simulink model "publish_vector3"  (R2020a)
settings: Solver=ode3  StartTime=0.0  StopTime=inf  FixedStep=0.02  RelTol=1e-3
InitFcn:
  | ros_init_callback
undefined symbols (not defined in the file or in its folder): X, Y, Z
libraries: robotlib x3
settings Model: Creator=esl  LastModifiedBy=murray
settings OptimizationCC: EnhancedBackFolding=on  PassReuseOutputArgsAs=Individual arguments  ZeroExternalMemoryAtStartup=off  ZeroInternalMemoryAtStartup=off  MaxStackSize=64  OptimizeBlockOrder=speed  DifferentSizesBufferReuse=on  OptimizationCustomize=off  EfficientTunableParamExpr=on
settings DebuggingCC: ParameterTunabilityLossMsg=error  SFMachineParentedDataDiag=error
settings HardwareCC: ProdBitPerPointer=32  ProdBitPerSizeT=32  ProdBitPerPtrDiffT=32  ProdLargestAtomicInteger=Long  ProdLargestAtomicFloat=Double  ProdWordSize=32  ProdHWDeviceType=ARM Compatible->ARM Cortex  UseEmbeddedCoderFeatures=off
settings SFSimCC: MATLABDynamicMemAlloc=off
settings RTWCC: SystemTargetFile=ert.tlc  HardwareBoard=Robot Operating System (ROS)  TemplateMakefile=ert_default_tmf  GenerateReport=on  Toolchain=Catkin  BuildConfiguration=Faster Runs  LaunchReport=on  TargetLang=C++
settings CodeAppCC: ForceParamTrailComments=on  OperatorAnnotations=on  SimulinkDataObjDesc=on  SFDataObjDesc=on  InsertBlockDesc=on
settings ERTTargetCC: SupportNonInlinedSFcns=on  ERTSrcFileBannerTemplate=codertarget_code_template.cgt  ERTHdrFileBannerTemplate=codertarget_code_template.cgt  ERTDataSrcFileTemplate=codertarget_code_template.cgt  ERTDataHdrFileTemplate=codertarget_code_template.cgt

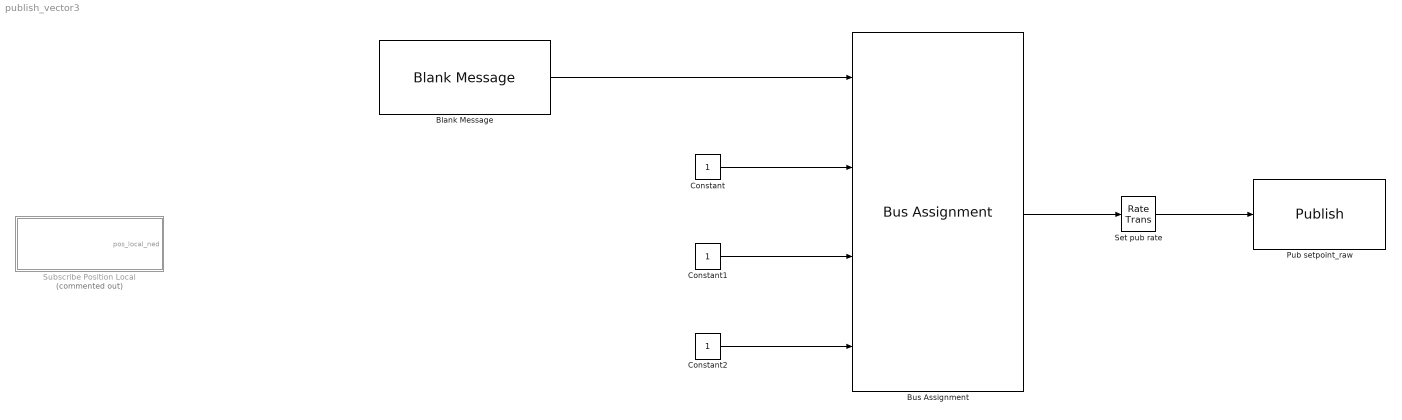
== system publish_vector3 ==
  Blank Message : robotlib/Blank Message  messageClass=Message  entityType=geometry_msgs/Vector3  messageType=geometry_msgs/Vector3  SampleTime=inf
  Bus Assignment : BusAssignment  AssignedSignals=X,Y,Z
  Constant : Constant
  Constant1 : Constant
  Constant2 : Constant
  Pub setpoint_raw : robotlib/Publish  topicSource=Specify your own  topic=/simulink/pos_sp  messageType=geometry_msgs/Vector3  messageQueueLength=1
  Set pub rate : RateTransition  OutPortSampleTime=0.01
  Subscribe Position Local : Subsystem  Commented=on
  wires:
  Blank Message/1 -> Bus Assignment/1
  Bus Assignment/1 -> Set pub rate/1
  Set pub rate/1 -> Pub setpoint_raw/1
  Constant/1 -> Bus Assignment/2
  Constant1/1 -> Bus Assignment/3
  Constant2/1 -> Bus Assignment/4

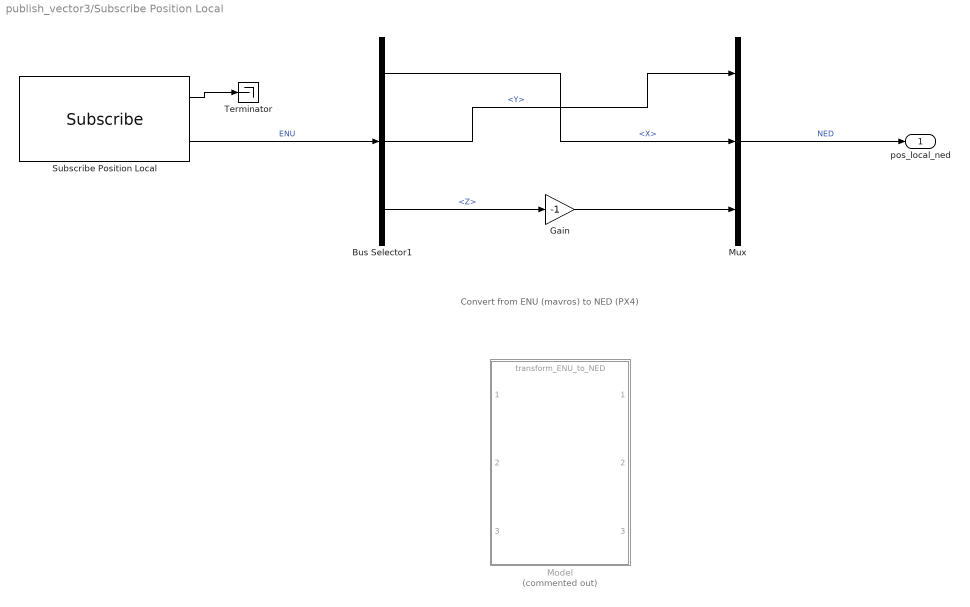
== system publish_vector3/Subscribe Position Local ==
  note: Convert from ENU (mavros) to NED (PX4)
  Bus Selector1 : BusSelector  OutputSignals=Pose.Position.X,Pose.Position.Y,Pose.Position.Z
  Gain : Gain  Gain=-1
  Model : ModelReference  Commented=on  ModelNameDialog=transform_ENU_to_NED.slx  SimulationMode=Normal  ModelReferenceVersion=1.10
  Mux : Mux  Inputs=3
  Subscribe Position Local : robotlib/Subscribe  topicSource=Select from ROS network  topic=/mavros/local_position/pose  messageType=geometry_msgs/PoseStamped  sampleTime=Ts_sub  messageQueueLength=1
  Terminator : Terminator
  pos_local_ned : Outport
  wires:
  Subscribe Position Local/1 -> Terminator/1
  Mux/1 -> pos_local_ned/1  "NED"
  Subscribe Position Local/2 -> Bus Selector1/1  "ENU"
  Bus Selector1/1 -> Mux/2  "<X>"
  Bus Selector1/2 -> Mux/1  "<Y>"
  Bus Selector1/3 -> Gain/1  "<Z>"
  Gain/1 -> Mux/3
